simulink subsystem "ADRC"  (R2022a)
settings: Solver=VariableStepAuto  StartTime=0.0  StopTime=10.0  RelTol=1e-3
model mask{para=0}
  mask prompts: para "控制器参数(结构体)"
undefined symbols (not defined in the file or in its folder): para_u
settings Model: Creator=45489  LastModifiedBy=45489

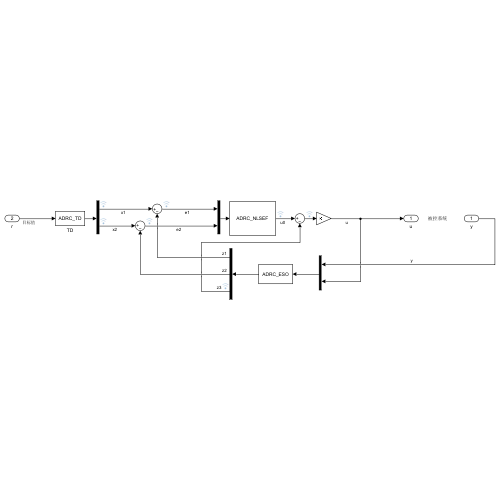
[thumbnail: Simulink's stored preview of the top-level diagram]
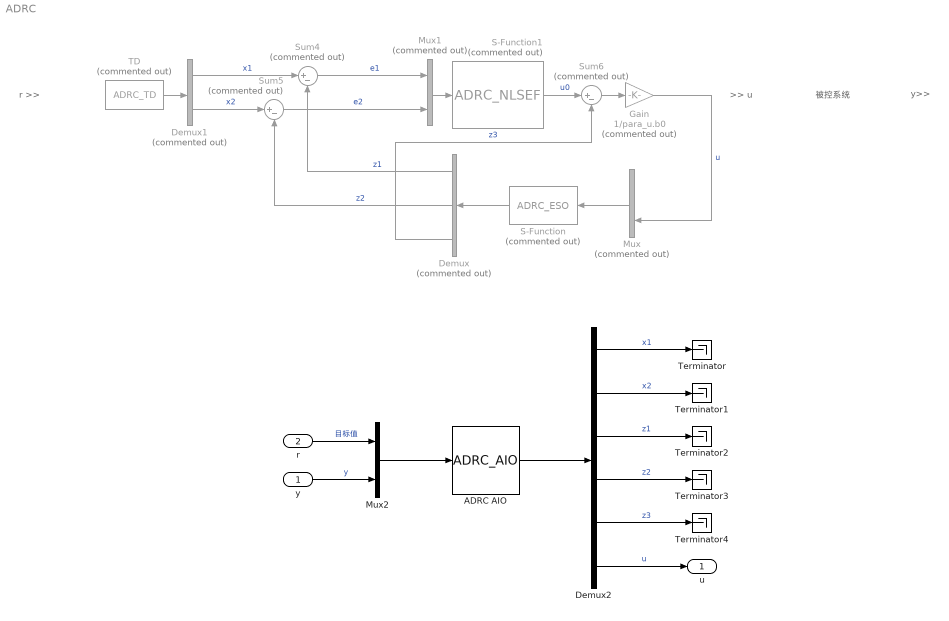
== system ADRC ==
  note: r >>
  note: y>>
  note: >> u
  note: 被控系统
  y : Inport
  r : Inport  Port=2
  ADRC AIO : S-Function  FunctionName=ADRC_AIO  Parameters=para  SFunctionDeploymentMode=off  EnableBusSupport=off
  Demux : Demux  Commented=on  Outputs=3
  Demux1 : Demux  Commented=on  Outputs=2
  Demux2 : Demux  Outputs=6
  Gain : Gain  Commented=on  Gain=1/para_u.b0
  Mux : Mux  Commented=on  Inputs=2
  Mux1 : Mux  Commented=on  Inputs=2
  Mux2 : Mux  Inputs=2
  S-Function : S-Function  Commented=on  FunctionName=ADRC_ESO  Parameters=para  SFunctionDeploymentMode=off  EnableBusSupport=off
  S-Function1 : S-Function  Commented=on  FunctionName=ADRC_NLSEF  Parameters=para  SFunctionDeploymentMode=off  EnableBusSupport=off
  Sum4 : Sum  Commented=on  Inputs=|+-
  Sum5 : Sum  Commented=on  Inputs=|+-
  Sum6 : Sum  Commented=on  Inputs=|+-
  TD : S-Function  Commented=on  FunctionName=ADRC_TD  Parameters=para  SFunctionDeploymentMode=off  EnableBusSupport=off
  Terminator{,1..4} (5 alike) : Terminator
  u : Outport
  wires:
  TD/1 -> Demux1/1
  Gain/1 -> Mux/2  "u"
  Mux/1 -> S-Function/1
  S-Function/1 -> Demux/1
  Demux1/1 -> Sum4/1  "x1"
  Sum6/1 -> Gain/1
  Demux1/2 -> Sum5/1  "x2"
  Demux/2 -> Sum5/2  "z2"
  Sum4/1 -> Mux1/1  "e1"
  Demux/3 -> Sum6/2  "z3"
  Demux/1 -> Sum4/2  "z1"
  Mux1/1 -> S-Function1/1
  Sum5/1 -> Mux1/2  "e2"
  S-Function1/1 -> Sum6/1  "u0"
  Mux2/1 -> ADRC AIO/1
  r/1 -> Mux2/1  "目标值"
  y/1 -> Mux2/2  "y"
  ADRC AIO/1 -> Demux2/1
  Demux2/6 -> u/1  "u"
  Demux2/1 -> Terminator/1  "x1"
  Demux2/2 -> Terminator1/1  "x2"
  Demux2/3 -> Terminator2/1  "z1"
  Demux2/4 -> Terminator3/1  "z2"
  Demux2/5 -> Terminator4/1  "z3"
